simulink subsystem "VehicleBody1DOFLongitudinalSSC"  (R2023a)
settings: Solver=VariableStepAuto  StartTime=0.0  StopTime=10.0  RelTol=1e-3
undefined symbols (not defined in the file): EnvGrvty, PlntVehCGHgtAxl, PlntWhlLdRadius
libraries: nesl_utility_internal x3, sdl_lib x1
settings Model: ModifiedByFormat=The MathWorks, Inc.  Creator=The MathWorks, Inc.  LastModifiedBy=The MathWorks, Inc.
settings OptimizationCC: ReuseModelBlockBuffer=off

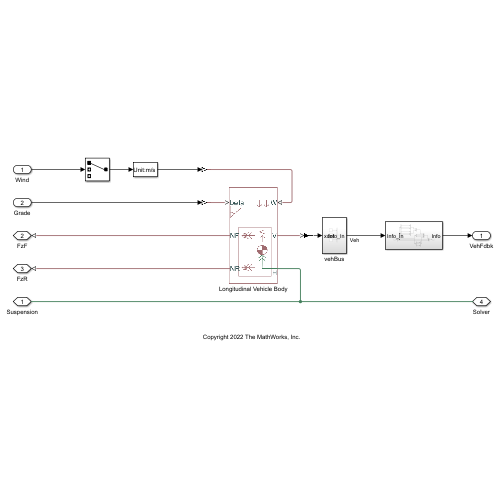
[thumbnail: Simulink's stored preview of the top-level diagram]
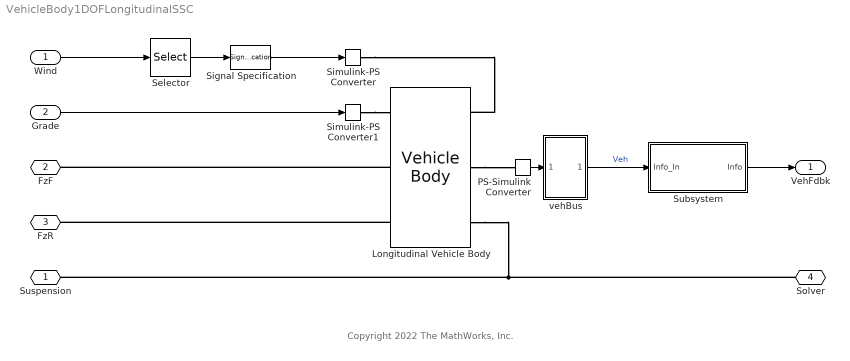
== system VehicleBody1DOFLongitudinalSSC ==
  note: Copyright 2022 The MathWorks, Inc.
  Wind : Inport  Unit=m/s
  Grade : Inport  Port=2  Unit=deg
  Longitudinal Vehicle Body : sdl_lib/Tires & Vehicles/Vehicle Body  mass=PlntVehMass kg  n_w=PlntVehNumWhlFrntAxl  x_f=PlntVehDstCGFrntAxl m  x_r=PlntVehDstCGRearAxl m  y_c=PlntVehCGHgtAxl+PlntWhlLdRadius m  mass_var=simscape.enum.onoff.off  g=EnvGrvty m/s^2  liftoff_warning=simscape.enum.onoff.off  area=PlntVehAeroFrntArea m^2  Cd=PlntVehAeroDragCff  rho=EnvAirDen kg/m^3  model_pitch=simscape.enum.onoff.off  inertia=4000 kg*m^2  suspension_model=sdl.enum.linearTLU.linear  k_f=1e4 N/m  b_f=1e4 N*s/m  k_r=1e4 N/m  b_r=1e4 N*s/m  k_f_TLU=[-2000, -1000, 0, 1000, 2000] N  x_f_TLU=[-.4, -.2, 0, .2, .4] m  b_f_TLU=[-200, -100, 0, 100, 200] N  v_f_TLU=[-4, -2, 0, 2, 4] m/s  k_r_TLU=[-2000, -1000, 0, 1000, 2000] N  x_r_TLU=[-.4, -.2, 0, .2, .4] m  b_r_TLU=[-200, -100, 0, 100, 200] N  v_r_TLU=[-4, -2, 0, 2, 4] m/s  interp_method=simscape.enum.interpolation.linear  extrap_method=simscape.enum.extrapolation.linear  model_hardstop=simscape.enum.onoff.off  upper_bound_f=.25 m  lower_bound_f=-.25 m  stop_k_f=1e6 N/m  stop_b_f=150 N*s/m  upper_bound_r=.25 m  lower_bound_r=-.25 m  stop_k_r=1e6 N/m  stop_b_r=150 N*s/m  initial_pitch=0 rad  initial_pitch_rate=0 rad/s  v_specify=off  v_priority=High  v=0 m/s  v_nominal_specify=off  v_nominal_unit=m/s  v_nominal_value=1
      settings: SourceProductName=Driveline
  PS-Simulink Converter : nesl_utility_internal/PS-Simulink Converter  PhysicalDomain=network_engine_domain  SubClassName=ps_output  LeftPortType=input  RightPortType=output  PseudoPeriodic=off  Frequencies=[]  VectorFormat=inherit  Unit=inherit  AffineConversion=off
  Selector : Selector  InputPortWidth=3  IndexOptions=Index vector (dialog)  Indices=[1]  OutputSizes=1
  Signal Specification : SignalSpecification  Unit=m/s
  Simulink-PS Converter : nesl_utility_internal/Simulink-PS Converter  PhysicalDomain=network_engine_domain  SubClassName=ps_input  LeftPortType=input  RightPortType=output  PseudoPeriodic=off  Frequencies=[]  NoiseDistribution=none  NoiseParameters=[]  Unit=m/s  AffineConversion=off  FilteringAndDerivatives=provide  SimscapeFilterOrder=1  InputFilterTimeConstant=0.001  UdotUserProvided=0
  Simulink-PS Converter1 : nesl_utility_internal/Simulink-PS Converter  PhysicalDomain=network_engine_domain  SubClassName=ps_input  LeftPortType=input  RightPortType=output  PseudoPeriodic=off  Frequencies=[]  NoiseDistribution=none  NoiseParameters=[]  Unit=deg  AffineConversion=off  FilteringAndDerivatives=provide  SimscapeFilterOrder=1  InputFilterTimeConstant=0.001  UdotUserProvided=0
  Subsystem : Subsystem
  vehBus : Subsystem
  Suspension : PMIOPort  Side=Right
  FzF : PMIOPort  Port=2  Side=Right
  FzR : PMIOPort  Port=3  Side=Right
  Solver : PMIOPort  Port=4  Side=Right
  VehFdbk : Outport  VectorParamsAs1DForOutWhenUnconnected=off
  wires:
  Wind/1 -> Selector/1
  Subsystem/1(Info) -> VehFdbk/1
  Selector/1 -> Signal Specification/1
  Grade/1 -> Simulink-PS Converter1/1
  PS-Simulink Converter/1 -> vehBus/1(xdot)
  vehBus/1(Info_In) -> Subsystem/1(Info_In)  "Veh"
  Signal Specification/1 -> Simulink-PS Converter/1
  connections:
  Longitudinal Vehicle Body/LConn1 -- Solver/RConn1 -- Suspension/RConn1
  Simulink-PS Converter/RConn1 -- Longitudinal Vehicle Body/LConn3
  Longitudinal Vehicle Body/LConn2 -- PS-Simulink Converter/LConn1
  Simulink-PS Converter1/RConn1 -- Longitudinal Vehicle Body/RConn3
  Longitudinal Vehicle Body/RConn2 -- FzF/RConn1
  Longitudinal Vehicle Body/RConn1 -- FzR/RConn1

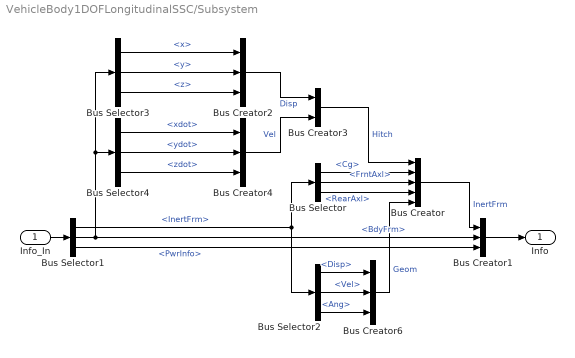
== system VehicleBody1DOFLongitudinalSSC/Subsystem ==
  Info_In : Inport
  Bus Creator : BusCreator  Inputs=5
  Bus Creator{1..2,4,6} (4 alike) : BusCreator  Inputs=3
  Bus Creator3 : BusCreator  Inputs=2
  Bus Selector : BusSelector  OutputSignals=Cg,FrntAxl,RearAxl
  Bus Selector1 : BusSelector  OutputSignals=InertFrm,BdyFrm,PwrInfo
  Bus Selector2 : BusSelector  OutputSignals=Cg.Disp,Cg.Vel,Cg.Ang
  Bus Selector3 : BusSelector  OutputSignals=Cg.Disp.x,Cg.Disp.y,Cg.Disp.z
  Bus Selector4 : BusSelector  OutputSignals=Cg.Vel.xdot,Cg.Vel.ydot,Cg.Vel.zdot
  Info : Outport
  wires:
  Bus Selector2/3 -> Bus Creator6/3  "<Ang>"
  Bus Selector2/2 -> Bus Creator6/2  "<Vel>"
  Bus Selector2/1 -> Bus Creator6/1  "<Disp>"
  Bus Creator6/1 -> Bus Creator/5  "Geom"
  Bus Selector1/2 -> Bus Creator1/2, Bus Selector3/1, Bus Selector4/1  "<BdyFrm>"
  Info_In/1 -> Bus Selector1/1
  Bus Creator/1 -> Bus Creator1/1  "InertFrm"
  Bus Selector/3 -> Bus Creator/4  "<RearAxl>"
  Bus Selector1/1 -> Bus Selector/1, Bus Selector2/1  "<InertFrm>"
  Bus Creator1/1 -> Info/1
  Bus Creator3/1 -> Bus Creator/1  "Hitch"
  Bus Selector1/3 -> Bus Creator1/3  "<PwrInfo>"
  Bus Selector/1 -> Bus Creator/2  "<Cg>"
  Bus Selector/2 -> Bus Creator/3  "<FrntAxl>"
  Bus Creator4/1 -> Bus Creator3/2  "Vel"
  Bus Creator2/1 -> Bus Creator3/1  "Disp"
  Bus Selector3/1 -> Bus Creator2/1  "<x>"
  Bus Selector3/2 -> Bus Creator2/2  "<y>"
  Bus Selector3/3 -> Bus Creator2/3  "<z>"
  Bus Selector4/1 -> Bus Creator4/1  "<xdot>"
  Bus Selector4/2 -> Bus Creator4/2  "<ydot>"
  Bus Selector4/3 -> Bus Creator4/3  "<zdot>"

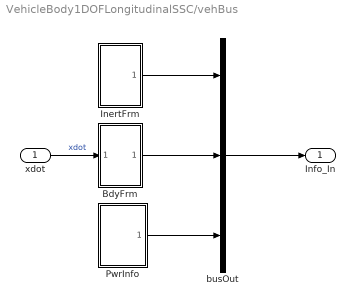
== system VehicleBody1DOFLongitudinalSSC/vehBus ==
  xdot : Inport
  BdyFrm : Subsystem
  InertFrm : Subsystem
  PwrInfo : Subsystem
  busOut : BusCreator  Inputs=3
  Info_In : Outport
  wires:
  busOut/1 -> Info_In/1
  PwrInfo/1(PwrInfo) -> busOut/3
  InertFrm/1(InertFrm) -> busOut/1
  BdyFrm/1(BdyFrm) -> busOut/2
  xdot/1 -> BdyFrm/1(xdot)  "xdot"

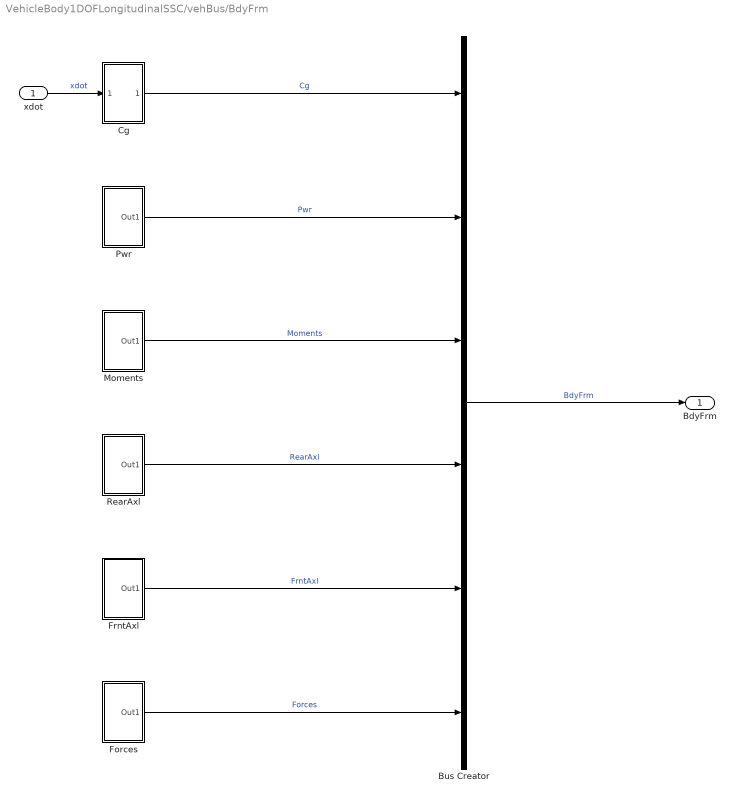
== system VehicleBody1DOFLongitudinalSSC/vehBus/BdyFrm ==
  xdot : Inport
  Bus Creator : BusCreator  Inputs=6
  Cg : Subsystem
  Forces : Subsystem
  FrntAxl : Subsystem
  Moments : Subsystem
  Pwr : Subsystem
  RearAxl : Subsystem
  BdyFrm : Outport
  wires:
  Bus Creator/1 -> BdyFrm/1  "BdyFrm"
  Pwr/1(Out1) -> Bus Creator/2  "Pwr"
  Moments/1(Out1) -> Bus Creator/3  "Moments"
  RearAxl/1(Out1) -> Bus Creator/4  "RearAxl"
  FrntAxl/1(Out1) -> Bus Creator/5  "FrntAxl"
  Forces/1(Out1) -> Bus Creator/6  "Forces"
  Cg/1(Out1) -> Bus Creator/1  "Cg"
  xdot/1 -> Cg/1(xdot)  "xdot"

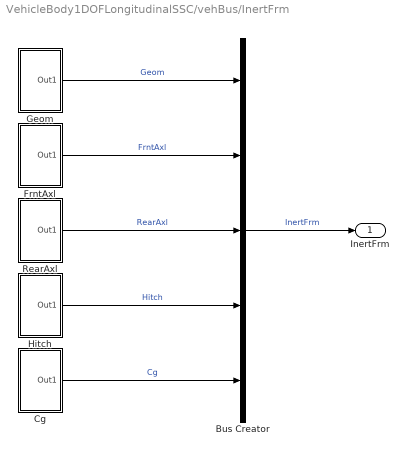
== system VehicleBody1DOFLongitudinalSSC/vehBus/InertFrm ==
  Bus Creator : BusCreator  Inputs=5
  Cg : Subsystem
  FrntAxl : Subsystem
  Geom : Subsystem
  Hitch : Subsystem
  RearAxl : Subsystem
  InertFrm : Outport
  wires:
  Bus Creator/1 -> InertFrm/1  "InertFrm"
  Cg/1(Out1) -> Bus Creator/5  "Cg"
  Geom/1(Out1) -> Bus Creator/1  "Geom"
  FrntAxl/1(Out1) -> Bus Creator/2  "FrntAxl"
  RearAxl/1(Out1) -> Bus Creator/3  "RearAxl"
  Hitch/1(Out1) -> Bus Creator/4  "Hitch"

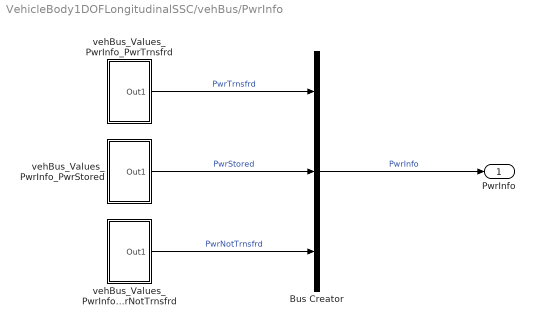
== system VehicleBody1DOFLongitudinalSSC/vehBus/PwrInfo ==
  Bus Creator : BusCreator  Inputs=3
  vehBus_Values_PwrInfo_PwrNotTrnsfrd : Subsystem
  vehBus_Values_PwrInfo_PwrStored : Subsystem
  vehBus_Values_PwrInfo_PwrTrnsfrd : Subsystem
  PwrInfo : Outport
  wires:
  vehBus_Values_PwrInfo_PwrTrnsfrd/1(Out1) -> Bus Creator/1  "PwrTrnsfrd"
  vehBus_Values_PwrInfo_PwrStored/1(Out1) -> Bus Creator/2  "PwrStored"
  vehBus_Values_PwrInfo_PwrNotTrnsfrd/1(Out1) -> Bus Creator/3  "PwrNotTrnsfrd"
  Bus Creator/1 -> PwrInfo/1  "PwrInfo"

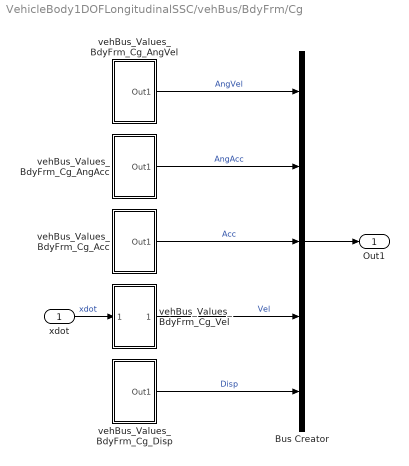
== system VehicleBody1DOFLongitudinalSSC/vehBus/BdyFrm/Cg ==
  xdot : Inport
  Bus Creator : BusCreator  Inputs=5
  vehBus_Values_BdyFrm_Cg_Acc : Subsystem
  vehBus_Values_BdyFrm_Cg_AngAcc : Subsystem
  vehBus_Values_BdyFrm_Cg_AngVel : Subsystem
  vehBus_Values_BdyFrm_Cg_Disp : Subsystem
  vehBus_Values_BdyFrm_Cg_Vel : Subsystem
  Out1 : Outport
  wires:
  vehBus_Values_BdyFrm_Cg_Vel/1(Out1) -> Bus Creator/4  "Vel"
  vehBus_Values_BdyFrm_Cg_Disp/1(Out1) -> Bus Creator/5  "Disp"
  vehBus_Values_BdyFrm_Cg_AngVel/1(Out1) -> Bus Creator/1  "AngVel"
  vehBus_Values_BdyFrm_Cg_Acc/1(Out1) -> Bus Creator/3  "Acc"
  vehBus_Values_BdyFrm_Cg_AngAcc/1(Out1) -> Bus Creator/2  "AngAcc"
  Bus Creator/1 -> Out1/1
  xdot/1 -> vehBus_Values_BdyFrm_Cg_Vel/1(xdot)  "xdot"

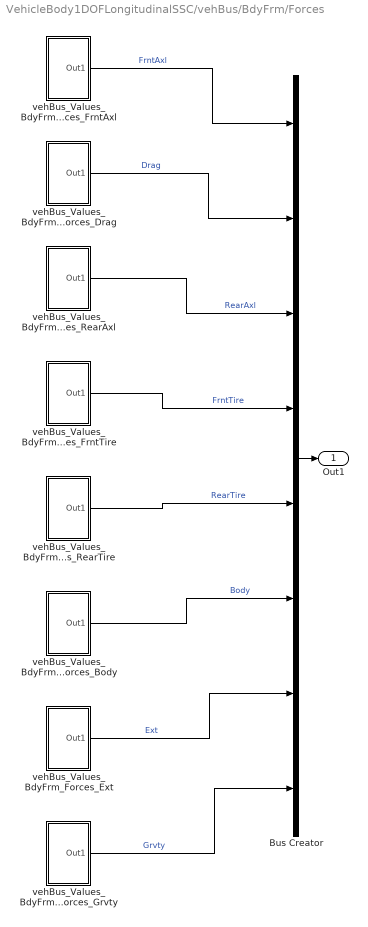
== system VehicleBody1DOFLongitudinalSSC/vehBus/BdyFrm/Forces ==
  Bus Creator : BusCreator  Inputs=8
  vehBus_Values_BdyFrm_Forces_Body : Subsystem
  vehBus_Values_BdyFrm_Forces_Drag : Subsystem
  vehBus_Values_BdyFrm_Forces_Ext : Subsystem
  vehBus_Values_BdyFrm_Forces_FrntAxl : Subsystem
  vehBus_Values_BdyFrm_Forces_Grvty : Subsystem
  vehBus_Values_BdyFrm_Forces_RearAxl : Subsystem
  vehBus_Values_BdyFrm_Forces_Tires_FrntTire : Subsystem
  vehBus_Values_BdyFrm_Forces_Tires_RearTire : Subsystem
  Out1 : Outport
  wires:
  vehBus_Values_BdyFrm_Forces_FrntAxl/1(Out1) -> Bus Creator/1  "FrntAxl"
  vehBus_Values_BdyFrm_Forces_Drag/1(Out1) -> Bus Creator/2  "Drag"
  vehBus_Values_BdyFrm_Forces_Grvty/1(Out1) -> Bus Creator/8  "Grvty"
  vehBus_Values_BdyFrm_Forces_Tires_RearTire/1(Out1) -> Bus Creator/5  "RearTire"
  vehBus_Values_BdyFrm_Forces_Body/1(Out1) -> Bus Creator/6  "Body"
  vehBus_Values_BdyFrm_Forces_Tires_FrntTire/1(Out1) -> Bus Creator/4  "FrntTire"
  vehBus_Values_BdyFrm_Forces_RearAxl/1(Out1) -> Bus Creator/3  "RearAxl"
  vehBus_Values_BdyFrm_Forces_Ext/1(Out1) -> Bus Creator/7  "Ext"
  Bus Creator/1 -> Out1/1

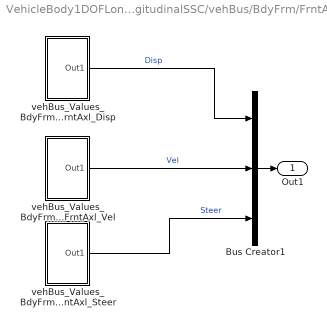
== system VehicleBody1DOFLongitudinalSSC/vehBus/BdyFrm/FrntAxl ==
  Bus Creator1 : BusCreator  Inputs=3
  vehBus_Values_BdyFrm_FrntAxl_Disp : Subsystem
  vehBus_Values_BdyFrm_FrntAxl_Steer : Subsystem
  vehBus_Values_BdyFrm_FrntAxl_Vel : Subsystem
  Out1 : Outport
  wires:
  vehBus_Values_BdyFrm_FrntAxl_Vel/1(Out1) -> Bus Creator1/2  "Vel"
  vehBus_Values_BdyFrm_FrntAxl_Steer/1(Out1) -> Bus Creator1/3  "Steer"
  vehBus_Values_BdyFrm_FrntAxl_Disp/1(Out1) -> Bus Creator1/1  "Disp"
  Bus Creator1/1 -> Out1/1

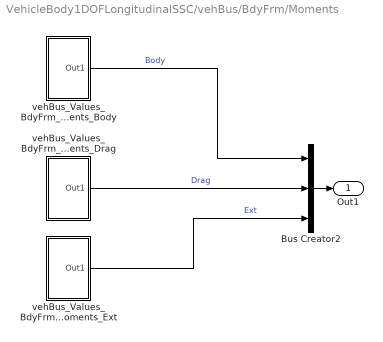
== system VehicleBody1DOFLongitudinalSSC/vehBus/BdyFrm/Moments ==
  Bus Creator2 : BusCreator  Inputs=3
  vehBus_Values_BdyFrm_Moments_Body : Subsystem
  vehBus_Values_BdyFrm_Moments_Drag : Subsystem
  vehBus_Values_BdyFrm_Moments_Ext : Subsystem
  Out1 : Outport
  wires:
  vehBus_Values_BdyFrm_Moments_Ext/1(Out1) -> Bus Creator2/3  "Ext"
  vehBus_Values_BdyFrm_Moments_Drag/1(Out1) -> Bus Creator2/2  "Drag"
  vehBus_Values_BdyFrm_Moments_Body/1(Out1) -> Bus Creator2/1  "Body"
  Bus Creator2/1 -> Out1/1

== system VehicleBody1DOFLongitudinalSSC/vehBus/BdyFrm/Pwr ==
  Drag : Constant  Value=zeros([1,1])
  PwrExt : Constant  Value=zeros([1,1])
  busOut : BusCreator  Inputs=2
  Out1 : Outport
  wires:
  busOut/1 -> Out1/1
  PwrExt/1 -> busOut/1  "PwrExt"
  Drag/1 -> busOut/2  "Drag"

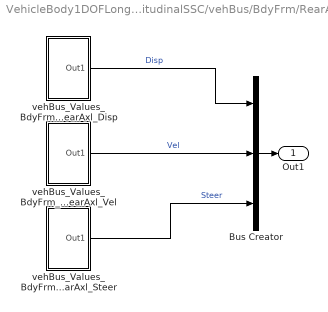
== system VehicleBody1DOFLongitudinalSSC/vehBus/BdyFrm/RearAxl ==
  Bus Creator : BusCreator  Inputs=3
  vehBus_Values_BdyFrm_RearAxl_Disp : Subsystem
  vehBus_Values_BdyFrm_RearAxl_Steer : Subsystem
  vehBus_Values_BdyFrm_RearAxl_Vel : Subsystem
  Out1 : Outport
  wires:
  Bus Creator/1 -> Out1/1
  vehBus_Values_BdyFrm_RearAxl_Steer/1(Out1) -> Bus Creator/3  "Steer"
  vehBus_Values_BdyFrm_RearAxl_Vel/1(Out1) -> Bus Creator/2  "Vel"
  vehBus_Values_BdyFrm_RearAxl_Disp/1(Out1) -> Bus Creator/1  "Disp"

== system VehicleBody1DOFLongitudinalSSC/vehBus/InertFrm/Cg ==
  Bus Creator4 : BusCreator  Inputs=3
  vehBus_Values_InertFrm_Cg_Ang : Subsystem
  vehBus_Values_InertFrm_Cg_Disp : Subsystem
  vehBus_Values_InertFrm_Cg_Vel : Subsystem
  Out1 : Outport
  wires:
  vehBus_Values_InertFrm_Cg_Disp/1(Out1) -> Bus Creator4/1  "Disp"
  vehBus_Values_InertFrm_Cg_Vel/1(Out1) -> Bus Creator4/2  "Vel"
  vehBus_Values_InertFrm_Cg_Ang/1(Out1) -> Bus Creator4/3  "Ang"
  Bus Creator4/1 -> Out1/1

== system VehicleBody1DOFLongitudinalSSC/vehBus/InertFrm/FrntAxl ==
  Bus Creator : BusCreator  Inputs=2
  vehBus_Values_InertFrm_FrntAxl_Disp : Subsystem
  vehBus_Values_InertFrm_FrntAxl_Vel : Subsystem
  Out1 : Outport
  wires:
  vehBus_Values_InertFrm_FrntAxl_Disp/1(Out1) -> Bus Creator/1  "Disp"
  vehBus_Values_InertFrm_FrntAxl_Vel/1(Out1) -> Bus Creator/2  "Vel"
  Bus Creator/1 -> Out1/1

== system VehicleBody1DOFLongitudinalSSC/vehBus/InertFrm/Geom ==
  Bus Creator3 : BusCreator  Inputs=3
  vehBus_Values_InertFrm_Geom_Ang : Subsystem
  vehBus_Values_InertFrm_Geom_Disp : Subsystem
  vehBus_Values_InertFrm_Geom_Vel : Subsystem
  Out1 : Outport
  wires:
  Bus Creator3/1 -> Out1/1
  vehBus_Values_InertFrm_Geom_Vel/1(Out1) -> Bus Creator3/2  "Vel"
  vehBus_Values_InertFrm_Geom_Ang/1(Out1) -> Bus Creator3/3  "Ang"
  vehBus_Values_InertFrm_Geom_Disp/1(Out1) -> Bus Creator3/1  "Disp"

== system VehicleBody1DOFLongitudinalSSC/vehBus/InertFrm/Hitch ==
  Bus Creator2 : BusCreator  Inputs=2
  vehBus_Values_InertFrm_Hitch_Disp : Subsystem
  vehBus_Values_InertFrm_Hitch_Vel : Subsystem
  Out1 : Outport
  wires:
  vehBus_Values_InertFrm_Hitch_Disp/1(Out1) -> Bus Creator2/1  "Disp"
  vehBus_Values_InertFrm_Hitch_Vel/1(Out1) -> Bus Creator2/2  "Vel"
  Bus Creator2/1 -> Out1/1

== system VehicleBody1DOFLongitudinalSSC/vehBus/InertFrm/RearAxl ==
  Bus Creator1 : BusCreator  Inputs=2
  vehBus_Values_InertFrm_RearAxl_Disp : Subsystem
  vehBus_Values_InertFrm_RearAxl_Vel : Subsystem
  Out1 : Outport
  wires:
  vehBus_Values_InertFrm_RearAxl_Disp/1(Out1) -> Bus Creator1/1  "Disp"
  vehBus_Values_InertFrm_RearAxl_Vel/1(Out1) -> Bus Creator1/2  "Vel"
  Bus Creator1/1 -> Out1/1

== system VehicleBody1DOFLongitudinalSSC/vehBus/PwrInfo/vehBus_Values_PwrInfo_PwrNotTrnsfrd ==
  PwrFxDrag : Constant  Value=zeros([1,1])
  busOut : BusCreator  Inputs=1
  Out1 : Outport
  wires:
  PwrFxDrag/1 -> busOut/1  "PwrFxDrag"
  busOut/1 -> Out1/1

== system VehicleBody1DOFLongitudinalSSC/vehBus/PwrInfo/vehBus_Values_PwrInfo_PwrStored ==
  PwrStoredGrvty : Constant  Value=zeros([1,1])
  PwrStoredxdot : Constant  Value=zeros([1,1])
  busOut : BusCreator  Inputs=2
  Out1 : Outport
  wires:
  busOut/1 -> Out1/1
  PwrStoredGrvty/1 -> busOut/1  "PwrStoredGrvty"
  PwrStoredxdot/1 -> busOut/2  "PwrStoredxdot"

== system VehicleBody1DOFLongitudinalSSC/vehBus/PwrInfo/vehBus_Values_PwrInfo_PwrTrnsfrd ==
  PwrFwFx : Constant  Value=zeros([1,1])
  PwrFwRx : Constant  Value=zeros([1,1])
  PwrFxExt : Constant  Value=zeros([1,1])
  busOut : BusCreator  Inputs=3
  Out1 : Outport
  wires:
  PwrFwRx/1 -> busOut/3  "PwrFwRx"
  PwrFwFx/1 -> busOut/2  "PwrFwFx"
  PwrFxExt/1 -> busOut/1  "PwrFxExt"
  busOut/1 -> Out1/1

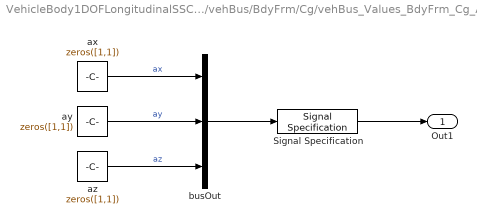
== system VehicleBody1DOFLongitudinalSSC/vehBus/BdyFrm/Cg/vehBus_Values_BdyFrm_Cg_Acc ==
  Signal Specification : SignalSpecification  Unit=m/s^2
  ax : Constant  Value=zeros([1,1])
  ay : Constant  Value=zeros([1,1])
  az : Constant  Value=zeros([1,1])
  busOut : BusCreator  Inputs=3
  Out1 : Outport
  wires:
  az/1 -> busOut/3  "az"
  ay/1 -> busOut/2  "ay"
  ax/1 -> busOut/1  "ax"
  busOut/1 -> Signal Specification/1
  Signal Specification/1 -> Out1/1

== system VehicleBody1DOFLongitudinalSSC/vehBus/BdyFrm/Cg/vehBus_Values_BdyFrm_Cg_AngAcc ==
  busOut : BusCreator  Inputs=3
  pdot : Constant  Value=zeros([1,1])
  qdot : Constant  Value=zeros([1,1])
  rdot : Constant  Value=zeros([1,1])
  Out1 : Outport
  wires:
  qdot/1 -> busOut/2  "qdot"
  pdot/1 -> busOut/1  "pdot"
  busOut/1 -> Out1/1
  rdot/1 -> busOut/3  "rdot"

== system VehicleBody1DOFLongitudinalSSC/vehBus/BdyFrm/Cg/vehBus_Values_BdyFrm_Cg_AngVel ==
  busOut : BusCreator  Inputs=3
  p : Constant  Value=zeros([1,1])
  q : Constant  Value=zeros([1,1])
  r : Constant  Value=zeros([1,1])
  Out1 : Outport
  wires:
  q/1 -> busOut/2  "q"
  busOut/1 -> Out1/1
  p/1 -> busOut/1  "p"
  r/1 -> busOut/3  "r"

== system VehicleBody1DOFLongitudinalSSC/vehBus/BdyFrm/Cg/vehBus_Values_BdyFrm_Cg_Disp ==
  busOut : BusCreator  Inputs=3
  x : Constant  Value=zeros([1,1])
  y : Constant  Value=zeros([1,1])
  z : Constant  Value=zeros([1,1])
  Out1 : Outport
  wires:
  busOut/1 -> Out1/1
  x/1 -> busOut/1  "x"
  y/1 -> busOut/2  "y"
  z/1 -> busOut/3  "z"

== system VehicleBody1DOFLongitudinalSSC/vehBus/BdyFrm/Cg/vehBus_Values_BdyFrm_Cg_Vel ==
  xdot : Inport
  busOut : BusCreator  Inputs=3
  ydot : Constant  Value=zeros([1,1])
  zdot : Constant  Value=zeros([1,1])
  Out1 : Outport
  wires:
  busOut/1 -> Out1/1
  ydot/1 -> busOut/2  "ydot"
  zdot/1 -> busOut/3  "zdot"
  xdot/1 -> busOut/1  "xdot"

== system VehicleBody1DOFLongitudinalSSC/vehBus/BdyFrm/Forces/vehBus_Values_BdyFrm_Forces_Body ==
  Fx : Constant  Value=zeros([1,1])
  Fy : Constant  Value=zeros([1,1])
  Fz : Constant  Value=zeros([1,1])
  busOut : BusCreator  Inputs=3
  Out1 : Outport
  wires:
  Fz/1 -> busOut/3  "Fz"
  Fx/1 -> busOut/1  "Fx"
  Fy/1 -> busOut/2  "Fy"
  busOut/1 -> Out1/1

== system VehicleBody1DOFLongitudinalSSC/vehBus/BdyFrm/Forces/vehBus_Values_BdyFrm_Forces_Drag ==
  Fx : Constant  Value=zeros([1,1])
  Fy : Constant  Value=zeros([1,1])
  Fz : Constant  Value=zeros([1,1])
  busOut : BusCreator  Inputs=3
  Out1 : Outport
  wires:
  busOut/1 -> Out1/1
  Fy/1 -> busOut/2  "Fy"
  Fx/1 -> busOut/1  "Fx"
  Fz/1 -> busOut/3  "Fz"

== system VehicleBody1DOFLongitudinalSSC/vehBus/BdyFrm/Forces/vehBus_Values_BdyFrm_Forces_Ext ==
  Fx : Constant  Value=zeros([1,1])
  Fy : Constant  Value=zeros([1,1])
  Fz : Constant  Value=zeros([1,1])
  busOut : BusCreator  Inputs=3
  Out1 : Outport
  wires:
  Fz/1 -> busOut/3  "Fz"
  Fy/1 -> busOut/2  "Fy"
  busOut/1 -> Out1/1
  Fx/1 -> busOut/1  "Fx"

== system VehicleBody1DOFLongitudinalSSC/vehBus/BdyFrm/Forces/vehBus_Values_BdyFrm_Forces_FrntAxl ==
  Fx : Constant  Value=zeros([1,4526])
  Fy : Constant  Value=zeros([1,1])
  Fz : Constant  Value=zeros([1,1])
  busOut : BusCreator  Inputs=3
  Out1 : Outport
  wires:
  Fy/1 -> busOut/2  "Fy"
  busOut/1 -> Out1/1
  Fx/1 -> busOut/1  "Fx"
  Fz/1 -> busOut/3  "Fz"

== system VehicleBody1DOFLongitudinalSSC/vehBus/BdyFrm/Forces/vehBus_Values_BdyFrm_Forces_Grvty ==
  Fx : Constant  Value=zeros([1,1])
  Fy : Constant  Value=zeros([1,1])
  Fz : Constant  Value=zeros([1,1])
  busOut : BusCreator  Inputs=3
  Out1 : Outport
  wires:
  Fx/1 -> busOut/1  "Fx"
  Fy/1 -> busOut/2  "Fy"
  Fz/1 -> busOut/3  "Fz"
  busOut/1 -> Out1/1

== system VehicleBody1DOFLongitudinalSSC/vehBus/BdyFrm/Forces/vehBus_Values_BdyFrm_Forces_RearAxl ==
  Fx : Constant  Value=zeros([1,4526])
  Fy : Constant  Value=zeros([1,1])
  Fz : Constant  Value=zeros([1,1])
  busOut : BusCreator  Inputs=3
  Out1 : Outport
  wires:
  Fx/1 -> busOut/1  "Fx"
  Fy/1 -> busOut/2  "Fy"
  Fz/1 -> busOut/3  "Fz"
  busOut/1 -> Out1/1

== system VehicleBody1DOFLongitudinalSSC/vehBus/BdyFrm/Forces/vehBus_Values_BdyFrm_Forces_Tires_FrntTire ==
  Fx : Constant  Value=zeros([1,1])
  Fy : Constant  Value=zeros([1,1])
  Fz : Constant  Value=zeros([1,1])
  busOut : BusCreator  Inputs=3
  Out1 : Outport
  wires:
  Fx/1 -> busOut/1  "Fx"
  Fy/1 -> busOut/2  "Fy"
  Fz/1 -> busOut/3  "Fz"
  busOut/1 -> Out1/1

== system VehicleBody1DOFLongitudinalSSC/vehBus/BdyFrm/Forces/vehBus_Values_BdyFrm_Forces_Tires_RearTire ==
  Fx : Constant  Value=zeros([1,1])
  Fy : Constant  Value=zeros([1,1])
  Fz : Constant  Value=zeros([1,1])
  busOut : BusCreator  Inputs=3
  Out1 : Outport
  wires:
  Fx/1 -> busOut/1  "Fx"
  busOut/1 -> Out1/1
  Fz/1 -> busOut/3  "Fz"
  Fy/1 -> busOut/2  "Fy"

== system VehicleBody1DOFLongitudinalSSC/vehBus/BdyFrm/FrntAxl/vehBus_Values_BdyFrm_FrntAxl_Disp ==
  busOut : BusCreator  Inputs=3
  x : Constant  Value=zeros([1,1])
  y : Constant  Value=zeros([1,1])
  z : Constant  Value=zeros([1,1])
  Out1 : Outport
  wires:
  z/1 -> busOut/3  "z"
  x/1 -> busOut/1  "x"
  y/1 -> busOut/2  "y"
  busOut/1 -> Out1/1

== system VehicleBody1DOFLongitudinalSSC/vehBus/BdyFrm/FrntAxl/vehBus_Values_BdyFrm_FrntAxl_Steer ==
  WhlAngFL : Constant  Value=zeros([1,1])
  WhlAngFR : Constant  Value=zeros([1,1])
  busOut : BusCreator  Inputs=2
  Out1 : Outport
  wires:
  busOut/1 -> Out1/1
  WhlAngFR/1 -> busOut/2  "WhlAngFR"
  WhlAngFL/1 -> busOut/1  "WhlAngFL"

== system VehicleBody1DOFLongitudinalSSC/vehBus/BdyFrm/FrntAxl/vehBus_Values_BdyFrm_FrntAxl_Vel ==
  busOut : BusCreator  Inputs=3
  xdot : Constant  Value=zeros([1,1])
  ydot : Constant  Value=zeros([1,1])
  zdot : Constant  Value=zeros([1,1])
  Out1 : Outport
  wires:
  zdot/1 -> busOut/3  "zdot"
  xdot/1 -> busOut/1  "xdot"
  ydot/1 -> busOut/2  "ydot"
  busOut/1 -> Out1/1

== system VehicleBody1DOFLongitudinalSSC/vehBus/BdyFrm/Moments/vehBus_Values_BdyFrm_Moments_Body ==
  Mx : Constant  Value=zeros([1,1])
  My : Constant  Value=zeros([1,1])
  Mz : Constant  Value=zeros([1,1])
  busOut : BusCreator  Inputs=3
  Out1 : Outport
  wires:
  Mz/1 -> busOut/3  "Mz"
  My/1 -> busOut/2  "My"
  Mx/1 -> busOut/1  "Mx"
  busOut/1 -> Out1/1

== system VehicleBody1DOFLongitudinalSSC/vehBus/BdyFrm/Moments/vehBus_Values_BdyFrm_Moments_Drag ==
  Mx : Constant  Value=zeros([1,1])
  My : Constant  Value=zeros([1,1])
  Mz : Constant  Value=zeros([1,1])
  busOut : BusCreator  Inputs=3
  Out1 : Outport
  wires:
  Mx/1 -> busOut/1  "Mx"
  busOut/1 -> Out1/1
  Mz/1 -> busOut/3  "Mz"
  My/1 -> busOut/2  "My"

== system VehicleBody1DOFLongitudinalSSC/vehBus/BdyFrm/Moments/vehBus_Values_BdyFrm_Moments_Ext ==
  Mx : Constant  Value=zeros([1,1])
  My : Constant  Value=zeros([1,1])
  Mz : Constant  Value=zeros([1,1])
  busOut : BusCreator  Inputs=3
  Out1 : Outport
  wires:
  Mz/1 -> busOut/3  "Mz"
  My/1 -> busOut/2  "My"
  Mx/1 -> busOut/1  "Mx"
  busOut/1 -> Out1/1

== system VehicleBody1DOFLongitudinalSSC/vehBus/BdyFrm/RearAxl/vehBus_Values_BdyFrm_RearAxl_Disp ==
  busOut : BusCreator  Inputs=3
  x : Constant  Value=zeros([1,1])
  y : Constant  Value=zeros([1,1])
  z : Constant  Value=zeros([1,1])
  Out1 : Outport
  wires:
  z/1 -> busOut/3  "z"
  busOut/1 -> Out1/1
  y/1 -> busOut/2  "y"
  x/1 -> busOut/1  "x"

== system VehicleBody1DOFLongitudinalSSC/vehBus/BdyFrm/RearAxl/vehBus_Values_BdyFrm_RearAxl_Steer ==
  WhlAngRL : Constant  Value=zeros([1,1])
  WhlAngRR : Constant  Value=zeros([1,1])
  busOut : BusCreator  Inputs=2
  Out1 : Outport
  wires:
  WhlAngRR/1 -> busOut/2  "WhlAngRR"
  WhlAngRL/1 -> busOut/1  "WhlAngRL"
  busOut/1 -> Out1/1

== system VehicleBody1DOFLongitudinalSSC/vehBus/BdyFrm/RearAxl/vehBus_Values_BdyFrm_RearAxl_Vel ==
  busOut : BusCreator  Inputs=3
  xdot : Constant  Value=zeros([1,1])
  ydot : Constant  Value=zeros([1,1])
  zdot : Constant  Value=zeros([1,1])
  Out1 : Outport
  wires:
  busOut/1 -> Out1/1
  ydot/1 -> busOut/2  "ydot"
  zdot/1 -> busOut/3  "zdot"
  xdot/1 -> busOut/1  "xdot"

== system VehicleBody1DOFLongitudinalSSC/vehBus/InertFrm/Cg/vehBus_Values_InertFrm_Cg_Ang ==
  busOut : BusCreator  Inputs=3
  phi : Constant  Value=zeros([1,1])
  psi : Constant  Value=zeros([1,1])
  theta : Constant  Value=zeros([1,1])
  Out1 : Outport
  wires:
  psi/1 -> busOut/3  "psi"
  theta/1 -> busOut/2  "theta"
  busOut/1 -> Out1/1
  phi/1 -> busOut/1  "phi"

== system VehicleBody1DOFLongitudinalSSC/vehBus/InertFrm/Cg/vehBus_Values_InertFrm_Cg_Disp ==
  X : Constant  Value=zeros([1,1])
  Y : Constant  Value=zeros([1,1])
  Z : Constant  Value=zeros([1,1])
  busOut : BusCreator  Inputs=3
  Out1 : Outport
  wires:
  X/1 -> busOut/1  "X"
  Y/1 -> busOut/2  "Y"
  Z/1 -> busOut/3  "Z"
  busOut/1 -> Out1/1

== system VehicleBody1DOFLongitudinalSSC/vehBus/InertFrm/Cg/vehBus_Values_InertFrm_Cg_Vel ==
  Xdot : Constant  Value=zeros([1,1])
  Ydot : Constant  Value=zeros([1,1])
  Zdot : Constant  Value=zeros([1,1])
  busOut : BusCreator  Inputs=3
  Out1 : Outport
  wires:
  Ydot/1 -> busOut/2  "Ydot"
  Zdot/1 -> busOut/3  "Zdot"
  Xdot/1 -> busOut/1  "Xdot"
  busOut/1 -> Out1/1

== system VehicleBody1DOFLongitudinalSSC/vehBus/InertFrm/FrntAxl/vehBus_Values_InertFrm_FrntAxl_Disp ==
  X : Constant  Value=zeros([1,1])
  Y : Constant  Value=zeros([1,1])
  Z : Constant  Value=zeros([1,1])
  busOut : BusCreator  Inputs=3
  Out1 : Outport
  wires:
  Z/1 -> busOut/3  "Z"
  Y/1 -> busOut/2  "Y"
  busOut/1 -> Out1/1
  X/1 -> busOut/1  "X"

== system VehicleBody1DOFLongitudinalSSC/vehBus/InertFrm/FrntAxl/vehBus_Values_InertFrm_FrntAxl_Vel ==
  Xdot : Constant  Value=zeros([1,1])
  Ydot : Constant  Value=zeros([1,1])
  Zdot : Constant  Value=zeros([1,1])
  busOut : BusCreator  Inputs=3
  Out1 : Outport
  wires:
  Xdot/1 -> busOut/1  "Xdot"
  Zdot/1 -> busOut/3  "Zdot"
  Ydot/1 -> busOut/2  "Ydot"
  busOut/1 -> Out1/1

== system VehicleBody1DOFLongitudinalSSC/vehBus/InertFrm/Geom/vehBus_Values_InertFrm_Geom_Ang ==
  busOut : BusCreator  Inputs=3
  phi : Constant  Value=zeros([1,1])
  psi : Constant  Value=zeros([1,1])
  theta : Constant  Value=zeros([1,1])
  Out1 : Outport
  wires:
  theta/1 -> busOut/2  "theta"
  psi/1 -> busOut/3  "psi"
  phi/1 -> busOut/1  "phi"
  busOut/1 -> Out1/1

== system VehicleBody1DOFLongitudinalSSC/vehBus/InertFrm/Geom/vehBus_Values_InertFrm_Geom_Disp ==
  X : Constant  Value=zeros([1,1])
  Y : Constant  Value=zeros([1,1])
  Z : Constant  Value=zeros([1,1])
  busOut : BusCreator  Inputs=3
  Out1 : Outport
  wires:
  X/1 -> busOut/1  "X"
  Y/1 -> busOut/2  "Y"
  Z/1 -> busOut/3  "Z"
  busOut/1 -> Out1/1

== system VehicleBody1DOFLongitudinalSSC/vehBus/InertFrm/Geom/vehBus_Values_InertFrm_Geom_Vel ==
  Xdot : Constant  Value=zeros([1,1])
  Ydot : Constant  Value=zeros([1,1])
  Zdot : Constant  Value=zeros([1,1])
  busOut : BusCreator  Inputs=3
  Out1 : Outport
  wires:
  Xdot/1 -> busOut/1  "Xdot"
  Zdot/1 -> busOut/3  "Zdot"
  Ydot/1 -> busOut/2  "Ydot"
  busOut/1 -> Out1/1

== system VehicleBody1DOFLongitudinalSSC/vehBus/InertFrm/Hitch/vehBus_Values_InertFrm_Hitch_Disp ==
  X : Constant  Value=zeros([1,1])
  Y : Constant  Value=zeros([1,1])
  Z : Constant  Value=zeros([1,1])
  busOut : BusCreator  Inputs=3
  Out1 : Outport
  wires:
  busOut/1 -> Out1/1
  Y/1 -> busOut/2  "Y"
  X/1 -> busOut/1  "X"
  Z/1 -> busOut/3  "Z"

== system VehicleBody1DOFLongitudinalSSC/vehBus/InertFrm/Hitch/vehBus_Values_InertFrm_Hitch_Vel ==
  Xdot : Constant  Value=zeros([1,1])
  Ydot : Constant  Value=zeros([1,1])
  Zdot : Constant  Value=zeros([1,1])
  busOut : BusCreator  Inputs=3
  Out1 : Outport
  wires:
  Zdot/1 -> busOut/3  "Zdot"
  busOut/1 -> Out1/1
  Ydot/1 -> busOut/2  "Ydot"
  Xdot/1 -> busOut/1  "Xdot"

== system VehicleBody1DOFLongitudinalSSC/vehBus/InertFrm/RearAxl/vehBus_Values_InertFrm_RearAxl_Disp ==
  X : Constant  Value=zeros([1,1])
  Y : Constant  Value=zeros([1,1])
  Z : Constant  Value=zeros([1,1])
  busOut : BusCreator  Inputs=3
  Out1 : Outport
  wires:
  Y/1 -> busOut/2  "Y"
  X/1 -> busOut/1  "X"
  Z/1 -> busOut/3  "Z"
  busOut/1 -> Out1/1

== system VehicleBody1DOFLongitudinalSSC/vehBus/InertFrm/RearAxl/vehBus_Values_InertFrm_RearAxl_Vel ==
  Xdot : Constant  Value=zeros([1,1])
  Ydot : Constant  Value=zeros([1,1])
  Zdot : Constant  Value=zeros([1,1])
  busOut : BusCreator  Inputs=3
  Out1 : Outport
  wires:
  Zdot/1 -> busOut/3  "Zdot"
  Xdot/1 -> busOut/1  "Xdot"
  Ydot/1 -> busOut/2  "Ydot"
  busOut/1 -> Out1/1
